simulink model "System_3"  (R2022b)
settings: Solver=VariableStepAuto  StartTime=0.0  StopTime=10.0  MaxStep=1e-4  RelTol=1e-3
settings Model: Creator=Dongr  LastModifiedBy=Dongr

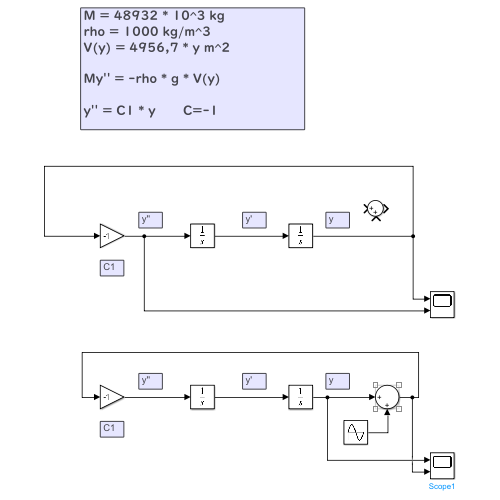
[thumbnail: Simulink's stored preview of the top-level diagram]
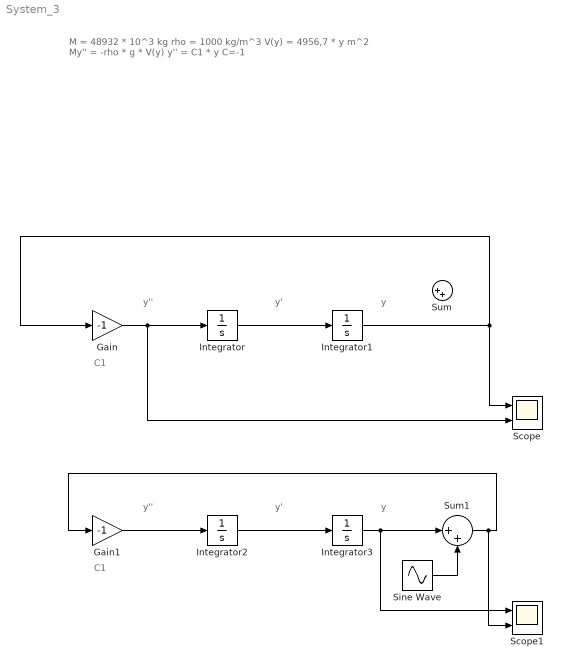
== system System_3 ==
  note: M = 48932 * 10^3 kg
      | rho = 1000 kg/m^3
      | V(y) = 4956,7 * y m^2
      |
      | My'' = -rho * g * V(y)
      |
      | y'' = C1 * y       C=-1
  note: C1
  note: y''
  note: y'
  note: y
  note: C1
  note: y''
  note: y'
  note: y
  Gain : Gain  Gain=-1
  Gain1 : Gain  Gain=-1
  Integrator : Integrator
  Integrator1 : Integrator  InitialCondition=1.5
  Integrator2 : Integrator
  Integrator3 : Integrator  InitialCondition=1.5
  Scope : Scope  NumInputPorts=2
  Scope1 : Scope  NumInputPorts=2
  Sine Wave : Sin  SampleTime=0
  Sum : Sum  Inputs=|++
  Sum1 : Sum  Inputs=|++
  wires:
  Integrator/1 -> Integrator1/1
  Gain/1 -> Scope/2, Integrator/1
  Integrator1/1 -> Scope/1, Gain/1
  Gain1/1 -> Integrator2/1
  Integrator2/1 -> Integrator3/1
  Integrator3/1 -> Sum1/1, Scope1/1
  Sum1/1 -> Scope1/2, Gain1/1
  Sine Wave/1 -> Sum1/2
